simulink model "analysis"  (R2020b)
settings: Solver=ode4  StartTime=0.0  StopTime=2  FixedStep=0.0001  RelTol=1e-3
libraries: sharedtransform x2, shared6dof x1, uavutilslib x1
settings Model: SimulationMode=accelerator  Creator=kcx06  LastModifiedBy=kcx06
settings DataIOCC: SaveOutput=off  DSMLogging=off  SaveTime=off

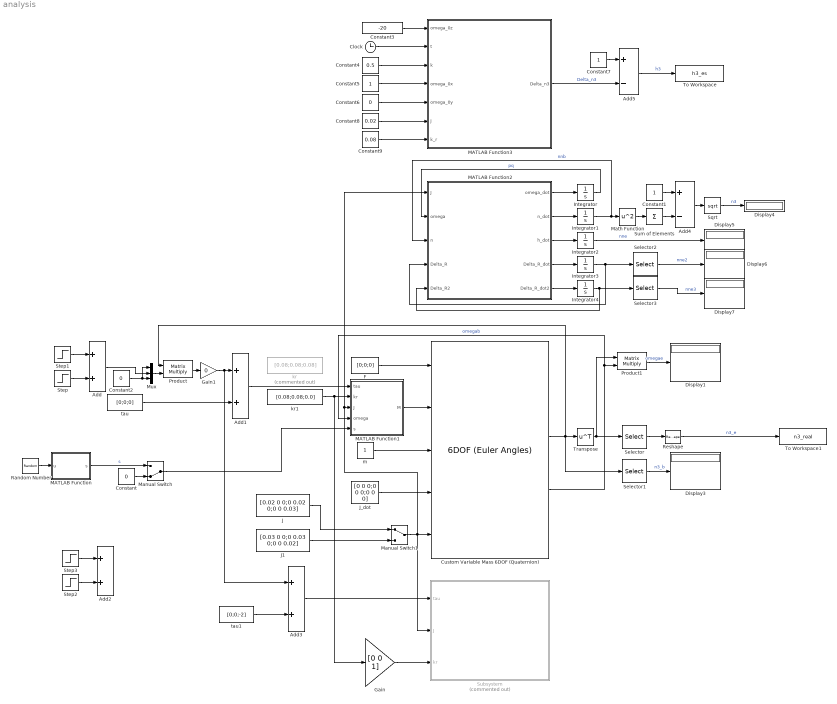
== system analysis ==
  Add{,1..3} (4 alike) : Sum
  Add4 : Sum  Inputs=+-
  Add5 : Sum  Inputs=+-
  Clock : Clock
  Constant : Constant  Value=0
  Constant1 : Constant
  Constant2 : Constant  Value=0
  Constant3 : Constant  Value=-20
  Constant4 : Constant  Value=0.5
  Constant5 : Constant
  Constant6 : Constant  Value=0
  Constant7 : Constant
  Constant8 : Constant  Value=0.02
  Constant9 : Constant  Value=0.08
  Custom Variable Mass 6DOF (Quaternion) : shared6dof/6DOF (Euler Angles)  units=Metric (MKS)  mtype=Custom Variable  rep=Quaternion  xme_0=[0 0 0]  Vm_0=[0 0 0]  eul_0=[0 0 0]  pm_0=[1 0 -20]  mass_0=1.0  mass_e=0.5  mass_f=2.0  inertia=eye(3)  inertia_e=eye(3)  inertia_f=2*eye(3)  k_quat=1.0  vre_flag=off  abi_flag=off  aMode=0  xme_statename=''  Vm_statename=''  eul_statename=''  quat_statename=''  pm_statename=''  mass_statename=''
      settings: SourceProductBaseCode=AE,PW,MT,UV,VE,VP
  Display{1,3..7} (6 alike) : Display
  F : Constant  Value=[0;0;0]
  Gain : Gain  Gain=[0 0 1]
  Gain1 : Gain  Gain=0
  Integrator : Integrator  InitialCondition=[1;0]
  Integrator1 : Integrator  InitialCondition=[0;0]
  Integrator2 : Integrator  InitialCondition=[0;0]
  Integrator3 : Integrator  InitialCondition=[0 0 0;0 0 0;0 0 0]
  Integrator4 : Integrator  InitialCondition=[0 0 0;0 0 0;0 0 0]
  J : Constant  Value=[0.02 0 0;0 0.02 0;0 0 0.03]
  J1 : Constant  Value=[0.03 0 0;0 0.03 0;0 0 0.02]
  J_dot : Constant  Value=[0 0 0;0 0 0;0 0 0]
  MATLAB Function : MATLAB Function  TreatAsAtomicUnit=on
  MATLAB Function1 : MATLAB Function  TreatAsAtomicUnit=on
  MATLAB Function2 : MATLAB Function  TreatAsAtomicUnit=on
  MATLAB Function3 : MATLAB Function  TreatAsAtomicUnit=on
  Manual Switch : ManualSwitch  CurrentSetting=0
  Manual Switch1 : ManualSwitch
  Math Function : Math  Operator=square  SaturateOnIntegerOverflow=on
  Mux : Mux  Inputs=3
  Product : Product  Multiplication=Matrix(*)
  Product1 : Product  Multiplication=Matrix(*)
  Random Number : RandomNumber  Seed=20  SampleTime=0.1
  Reshape : Reshape
  Selector{,1..3} (4 alike) : Selector  NumberOfDimensions=2  InputPortWidth=3  IndexOptions=Select all,Index vector (dialog)  Indices=[1 3],3  OutputSizes=1,1
  Sqrt : Sqrt  SaturateOnIntegerOverflow=on
  Step : Step  Time=5.001  After=-50  SampleTime=0.001
  Step1 : Step  Time=5  After=50  SampleTime=0.001
  Step2 : Step  Time=6.02  After=-1  SampleTime=0.001
  Step3 : Step  Time=6  SampleTime=0.001
  Subsystem : Subsystem  Commented=on
  Sum of Elements : Sum  Inputs=+
  To Workspace : ToWorkspace  VariableName=h3_es  SaveFormat=Timeseries  SampleTime=-1
  To Workspace1 : ToWorkspace  VariableName=n3_real  SaveFormat=Timeseries  SampleTime=-1
  Transpose : Math  Operator=transpose  SaturateOnIntegerOverflow=on
  kr : Constant  Commented=on  Value=[0.08;0.08;0.08]
  kr1 : Constant  Value=[0.08;0.08;0.0]
  m : Constant
  tau : Constant  Value=[0;0;0]
  tau1 : Constant  Value=[0;0;-2]
  wires:
  Manual Switch1/1 -> MATLAB Function2/1(J), MATLAB Function1/3(J), Subsystem/2(J), Custom Variable Mass 6DOF (Quaternion)/5
  tau/1 -> Add1/2
  kr1/1 -> Gain/1, MATLAB Function1/2(kr)
  Step1/1 -> Add/1
  Step/1 -> Add/2
  Constant2/1 -> Mux/1, Mux/3
  Mux/1 -> Product/2
  Add1/1 -> MATLAB Function1/1(tau)
  m/1 -> Custom Variable Mass 6DOF (Quaternion)/3
  J_dot/1 -> Custom Variable Mass 6DOF (Quaternion)/4
  F/1 -> Custom Variable Mass 6DOF (Quaternion)/1
  Custom Variable Mass 6DOF (Quaternion)/6 -> MATLAB Function1/4(omega), Product1/2  "omegab"
  MATLAB Function1/1(M) -> Custom Variable Mass 6DOF (Quaternion)/2
  Custom Variable Mass 6DOF (Quaternion)/4 -> Selector1/1, Product/1, Transpose/1
  Transpose/1 -> Product1/1, Selector/1
  Selector/1 -> Reshape/1
  Product1/1 -> Display1/1  "omegae"
  Manual Switch/1 -> MATLAB Function1/5(s)
  Step2/1 -> Add2/2
  Step3/1 -> Add2/1
  Constant/1 -> Manual Switch/2
  Add3/1 -> Subsystem/1(tau)
  Gain/1 -> Subsystem/3(kr)
  tau1/1 -> Add3/2
  Gain1/1 -> Add3/1, Add1/1
  Random Number/1 -> MATLAB Function/1(u)
  MATLAB Function/1(s) -> Manual Switch/1  "s"
  Selector1/1 -> Display3/1  "n3_b"
  J/1 -> Manual Switch1/1
  J1/1 -> Manual Switch1/2
  Add/1 -> Mux/2
  Product/1 -> Gain1/1
  MATLAB Function2/1(omega_dot) -> Integrator/1
  Integrator/1 -> MATLAB Function2/2(omega)  "pq"
  MATLAB Function2/2(n_dot) -> Integrator1/1
  Integrator1/1 -> Math Function/1, MATLAB Function2/3(n)  "nnb"
  Sum of Elements/1 -> Add4/2
  MATLAB Function2/3(h_dot) -> Integrator2/1
  Integrator2/1 -> Display5/1  "nne"
  MATLAB Function2/4(Delta_R_dot) -> Integrator3/1
  Integrator3/1 -> Selector2/1, MATLAB Function2/4(Delta_R)
  Selector2/1 -> Display6/1  "nne2"
  MATLAB Function2/5(Delta_R_dot2) -> Integrator4/1
  Integrator4/1 -> Selector3/1, MATLAB Function2/5(Delta_R2)
  Selector3/1 -> Display7/1  "nne3"
  Math Function/1 -> Sum of Elements/1
  Constant1/1 -> Add4/1
  Add4/1 -> Sqrt/1
  Sqrt/1 -> Display4/1  "n3"
  Constant3/1 -> MATLAB Function3/1(omega_0z)
  Clock/1 -> MATLAB Function3/2(t)
  Constant4/1 -> MATLAB Function3/3(k)
  Constant5/1 -> MATLAB Function3/4(omega_0x)
  Constant6/1 -> MATLAB Function3/5(omega_0y)
  MATLAB Function3/1(Delta_n3) -> Add5/2  "Delta_n3"
  Constant7/1 -> Add5/1
  Add5/1 -> To Workspace/1  "h3"
  Constant9/1 -> MATLAB Function3/7(k_r)
  Constant8/1 -> MATLAB Function3/6(J)
  Reshape/1 -> To Workspace1/1  "n3_e"

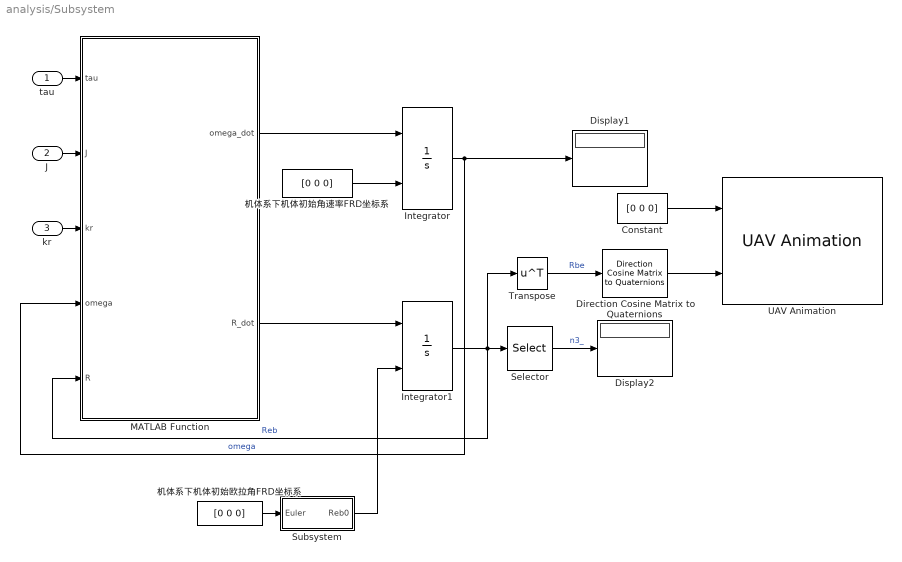
== system analysis/Subsystem ==
  tau : Inport
  J : Inport  Port=2
  kr : Inport  Port=3
  Constant : Constant  Value=[0 0 0]
  Direction Cosine Matrix to Quaternions : sharedtransform/Direction Cosine Matrix  to Quaternions  aMode=0  action=None  tolerance=eps(2)
      settings: SourceProductBaseCode=AE,PW,MT,UV,VE,VP
  Display1 : Display
  Display2 : Display
  Integrator : Integrator  InitialConditionSource=external  InitialCondition=[0;0;-19]
  Integrator1 : Integrator  InitialConditionSource=external  InitialCondition=[1 0 0;0 1 0;0 0 1]
  MATLAB Function : MATLAB Function  TreatAsAtomicUnit=on
  Selector : Selector  NumberOfDimensions=2  InputPortWidth=3  IndexOptions=Select all,Index vector (dialog)  Indices=[1 3],3  OutputSizes=1,1
  Subsystem : Subsystem
  Transpose : Math  Operator=transpose  SaturateOnIntegerOverflow=on
  UAV Animation : uavutilslib/UAV Animation  UAVType=Multirotor  UAVSize=1  InertialZDirection=Down  SampleTime=-1
      settings: SourceProductBaseCode=UV
  机体系下机体初始欧拉角FRD坐标系 : Constant  Value=[0 0 0]
  机体系下机体初始角速率FRD坐标系 : Constant  Value=[0 0 0]
  wires:
  MATLAB Function/1(omega_dot) -> Integrator/1
  tau/1 -> MATLAB Function/1(tau)
  Integrator/1 -> Display1/1, MATLAB Function/4(omega)  "omega"
  J/1 -> MATLAB Function/2(J)
  kr/1 -> MATLAB Function/3(kr)
  MATLAB Function/2(R_dot) -> Integrator1/1
  Integrator1/1 -> MATLAB Function/5(R), Transpose/1, Selector/1  "Reb"
  Selector/1 -> Display2/1  "n3_"
  Transpose/1 -> Direction Cosine Matrix to Quaternions/1  "Rbe"
  机体系下机体初始角速率FRD坐标系/1 -> Integrator/2
  机体系下机体初始欧拉角FRD坐标系/1 -> Subsystem/1(Euler)
  Subsystem/1(Reb0) -> Integrator1/2
  Constant/1 -> UAV Animation/1
  Direction Cosine Matrix to Quaternions/1 -> UAV Animation/2

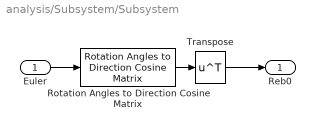
== system analysis/Subsystem/Subsystem ==
  Euler : Inport
  Rotation Angles to Direction Cosine Matrix : sharedtransform/Rotation Angles to Direction Cosine Matrix  rotationOrder=ZYX  aMode=aMode
      settings: SourceProductBaseCode=AE,PW,MT,UV,VE,VP
  Transpose : Math  Operator=transpose  SaturateOnIntegerOverflow=on
  Reb0 : Outport
  wires:
  Euler/1 -> Rotation Angles to Direction Cosine Matrix/1
  Rotation Angles to Direction Cosine Matrix/1 -> Transpose/1
  Transpose/1 -> Reb0/1

== matlab function analysis/MATLAB Function1 ==
  data: tau input; kr input; J input; M output; omega input; s input
function M = fcn(tau, kr, J, omega, s)
M = - kr.*omega + tau + s*cross(omega, J*omega);

== matlab function analysis/Subsystem/MATLAB Function ==
  data: tau input; omega_dot output; J input; kr input; omega input; R input; R_dot output
function [omega_dot, R_dot]= fcn(tau, J, kr, omega, R)

omega_dot = inv(J)*(-1*cross(omega, J*omega) - kr.*omega*norm(omega)  + tau);
% omega*norm(omega) 

R_dot = R*[0 -omega(3) omega(2); omega(3) 0 -omega(1); -omega(2) omega(1) 0];

== matlab function analysis/MATLAB Function ==
  data: u input; s output
function s = fcn(u)
if u>0
   s = 1.5; 
else
    s = 0;
end

== matlab function analysis/MATLAB Function2 ==
  data: J input; omega_dot output; omega input; n_dot output; n input; h_dot output; Delta_R input; Delta_R_dot output; Delta_R2 input; Delta_R_dot2 output
function [omega_dot, n_dot, h_dot, Delta_R_dot, Delta_R_dot2] = fcn(J, omega, n, Delta_R, Delta_R2)
omega_z0 = -20;
omega_x0 = 0;
omega_y0 = 0;
%omega_x等表示变化量
omega_x = omega(1);
omega_y = omega(2);
omega_z = 0;

omega_dot =1*[0 omega_z0*(J(2,2)-J(3,3))/J(1,1);...
                        omega_z0*(J(3,3)-J(1,1))/J(2,2)  0]*[omega(1);omega(2)];
%% 机体系下的n
n_dot = [0 omega_z0; -omega_z0 0]*n + [0 -1;1 0]*omega;
%%  
h_dot = [0 1;-1 0]*omega;
%% 考虑增量方程的四个项
Delta_R_dot = Delta_R*[0 -omega_z0 omega_y0; omega_z0 0 -omega_x0; -omega_y0 omega_x0 0] +...
    [0 -omega_z omega_y; omega_z 0 -omega_x; -omega_y omega_x 0] + ...
Delta_R*[0 -omega_z omega_y; omega_z 0 -omega_x; -omega_y omega_x 0] + ...
[0 -omega_z0 omega_y0; omega_z0 0 -omega_x0; -omega_y0 omega_x0 0];
%% 
Delta_R_dot2 = Delta_R2*[0 -omega_z0 omega_y; omega_z0 0 -omega_x; -omega_y omega_x 0] + [0 -omega_z0 omega_y; omega_z0 0 -omega_x; -omega_y omega_x 0];

== matlab function analysis/MATLAB Function3 ==
  data: omega_0z input; Delta_n3 output; t input; k input; omega_0x input; omega_0y input; J input; k_r input
function Delta_n3 = fcn(omega_0z,t,k,omega_0x,omega_0y, J, k_r)
k_rJ = k_r/J;
Delta_n3 =1/(2*(k^2*omega_0z^2 + 2*k*omega_0z^2 + k_rJ^2 + omega_0z^2))-...
    (exp((-2*k_rJ*t))*(2*exp((k_rJ*t))*cos(omega_0z*t*(k + 1)) - 1)*(omega_0x^2 + omega_0y^2))/(2*(k^2*omega_0z^2 + 2*k*omega_0z^2 + k_rJ^2 + omega_0z^2));
